simulink model "A1_VOO"  (R2020a)
settings: Solver=FixedStepAuto  StartTime=0.0  StopTime=10.0  FixedStep=1e-3  RelTol=1e-3  EnableMultiTasking=on
undefined symbols (not defined in the file): D10, D11, D12, D2, D4, D5, D7, D8, D9, PTA0, PTA2, PTB23, PTB9, PTC3, PTC4, PTD0, PTD2, PTD3
libraries: frdmk64flib x9
settings Model: ExtModeTrigDuration=5  Creator=Faisal  LastModifiedBy=Faisal
settings OptimizationCC: EnhancedBackFolding=on  PassReuseOutputArgsAs=Individual arguments  ZeroExternalMemoryAtStartup=off  ZeroInternalMemoryAtStartup=off  MaxStackSize=64  OptimizeBlockOrder=speed  DifferentSizesBufferReuse=on  OptimizationCustomize=off  EfficientTunableParamExpr=on
settings DebuggingCC: ParameterTunabilityLossMsg=error
settings HardwareCC: ProdBitPerPointer=32  ProdBitPerSizeT=32  ProdBitPerPtrDiffT=32  ProdLargestAtomicInteger=Long  ProdLargestAtomicFloat=Double  ProdWordSize=32  ProdHWDeviceType=ARM Compatible->ARM Cortex
settings SFSimCC: MATLABDynamicMemAlloc=off
settings RTWCC: SystemTargetFile=ert.tlc  HardwareBoard=NXP FRDM-K64F  TemplateMakefile=ert_default_tmf  Toolchain=GNU Tools for ARM Embedded Processors
settings CodeAppCC: ForceParamTrailComments=on  IgnoreCustomStorageClasses=off  OperatorAnnotations=on  SimulinkDataObjDesc=on  SFDataObjDesc=on  InsertBlockDesc=on

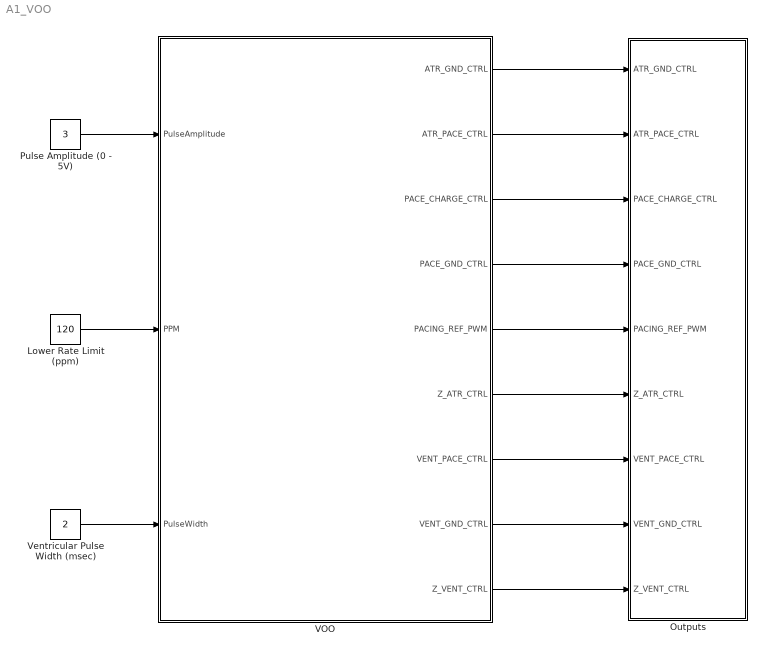
== system A1_VOO ==
  Lower Rate Limit (ppm) : Constant  Value=120  OutDataTypeStr=int16
  Outputs : Subsystem
  Pulse Amplitude (0 - 5V) : Constant  Value=3  OutDataTypeStr=double
  VOO : Stateflow chart  TreatAsAtomicUnit=on
  Ventricular Pulse Width (msec) : Constant  Value=2  OutDataTypeStr=double
  wires:
  Lower Rate Limit (ppm)/1 -> VOO/2(PPM)
  Pulse Amplitude (0 - 5V)/1 -> VOO/1(PulseAmplitude)
  Ventricular Pulse Width (msec)/1 -> VOO/3(PulseWidth)
  VOO/1(ATR_GND_CTRL) -> Outputs/1(ATR_GND_CTRL)
  VOO/2(ATR_PACE_CTRL) -> Outputs/2(ATR_PACE_CTRL)
  VOO/3(PACE_CHARGE_CTRL) -> Outputs/3(PACE_CHARGE_CTRL)
  VOO/4(PACE_GND_CTRL) -> Outputs/4(PACE_GND_CTRL)
  VOO/5(PACING_REF_PWM) -> Outputs/5(PACING_REF_PWM)
  VOO/6(Z_ATR_CTRL) -> Outputs/6(Z_ATR_CTRL)
  VOO/7(VENT_PACE_CTRL) -> Outputs/7(VENT_PACE_CTRL)
  VOO/8(VENT_GND_CTRL) -> Outputs/8(VENT_GND_CTRL)
  VOO/9(Z_VENT_CTRL) -> Outputs/9(Z_VENT_CTRL)

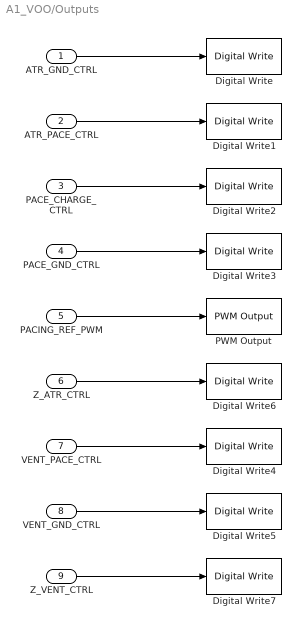
== system A1_VOO/Outputs ==
  ATR_GND_CTRL : Inport
  ATR_PACE_CTRL : Inport  Port=2
  PACE_CHARGE_CTRL : Inport  Port=3
  PACE_GND_CTRL : Inport  Port=4
  PACING_REF_PWM : Inport  Port=5
  Z_ATR_CTRL : Inport  Port=6
  VENT_PACE_CTRL : Inport  Port=7
  VENT_GND_CTRL : Inport  Port=8
  Z_VENT_CTRL : Inport  Port=9
  Digital Write : frdmk64flib/Digital Write  Whichpin=PTD2 (D11)
  Digital Write1 : frdmk64flib/Digital Write  Whichpin=PTA0 (D8)
  Digital Write2 : frdmk64flib/Digital Write  Whichpin=PTB9 (D2)
  Digital Write3 : frdmk64flib/Digital Write  Whichpin=PTD0 (D10)
  Digital Write4 : frdmk64flib/Digital Write  Whichpin=PTC4 (D9)
  Digital Write5 : frdmk64flib/Digital Write  Whichpin=PTD3 (D12)
  Digital Write6 : frdmk64flib/Digital Write  Whichpin=PTB23 (D4)
  Digital Write7 : frdmk64flib/Digital Write  Whichpin=PTC3 (D7)
  PWM Output : frdmk64flib/PWM Output  Whichpin=PTA2 (D5)  InitialFrequency=2000  InitialDutyCycle=100
  wires:
  PACE_CHARGE_CTRL/1 -> Digital Write2/1
  ATR_PACE_CTRL/1 -> Digital Write1/1
  VENT_PACE_CTRL/1 -> Digital Write4/1
  Z_VENT_CTRL/1 -> Digital Write7/1
  VENT_GND_CTRL/1 -> Digital Write5/1
  Z_ATR_CTRL/1 -> Digital Write6/1
  ATR_GND_CTRL/1 -> Digital Write/1
  PACE_GND_CTRL/1 -> Digital Write3/1
  PACING_REF_PWM/1 -> PWM Output/1

== stateflow chart A1_VOO/VOO ==
  state Charging_C22
    entry:
    %Charging C22
    ATR_PACE_CTRL=false;
    VENT_PACE_CTRL=false;
    PACING_REF_PWM = 20*PulseAmplitude;
    PACE_CHARGE_CTRL=true;
    %Discharging C21
    PACE_GND_CTRL=true;
    VENT_PACE_CTRL=false;
    Z_ATR_CTRL=false;
    Z_VENT_CTRL=false;
    ATR_GND_CTRL=false;
    VENT_GND_CTRL=true;
  state Pacing_Ventricle
    entry:
    %Discharging C22 into Ventricle
    PACE_CHARGE_CTRL=false;
    PACE_GND_CTRL=true;
    ATR_PACE_CTRL=false;
    ATR_GND_CTRL=false;
    Z_ATR_CTRL=false;
    Z_VENT_CTRL=false;
    VENT_GND_CTRL=false;
    VENT_PACE_CTRL=true;
  Pacing_Ventricle -> Charging_C22 : after(PulseWidth,msec)
  (default) -> Charging_C22
  Charging_C22 -> Pacing_Ventricle : after(((60000/PPM)-PulseWidth),msec)
  data: ATR_GND_CTRL output boolean; ATR_PACE_CTRL output boolean; PACE_CHARGE_CTRL output boolean; PACE_GND_CTRL output boolean; PACING_REF_PWM output double; Z_ATR_CTRL output boolean; PulseAmplitude input double; PPM input int16; PulseWidth input double; VENT_PACE_CTRL output boolean; VENT_GND_CTRL output boolean; Z_VENT_CTRL output boolean
